simulink model "N_v6_GUI"  (R2024b)
settings: Solver=FixedStepAuto  StartTime=0.0  StopTime=solvertime  FixedStep=stepsize  RelTol=1e-3
undefined symbols (not defined in the file or in its folder): phase_delay, pulse_amp, pulse_rate
libraries: Libs_unified x1
settings Model: Creator=ball907  LastModifiedBy=ball907
settings DataIOCC: ExternalInput=params

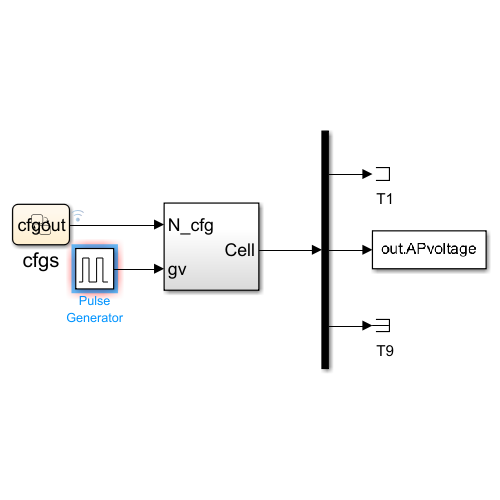
[thumbnail: Simulink's stored preview of the top-level diagram]
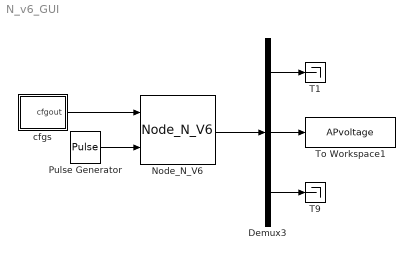
== system N_v6_GUI ==
  Demux3 : Demux  Outputs=[1, 1, 3]
  Node_N_V6 : Libs_unified/Node_N_V6  SystemSampleTime=-1  VariantActivationTime=update diagram  AllowFlexibleInterface=on  Latency=0  AutoFrameSizeCalculation=off
  Pulse Generator : DiscretePulseGenerator  PulseType=Time based  Amplitude=pulse_amp  Period=pulse_rate  PhaseDelay=phase_delay
  T1 : Terminator
  T9 : Terminator
  To Workspace1 : ToWorkspace  VariableName=APvoltage  SaveFormat=Timeseries  SampleTime=-1
  cfgs : Stateflow chart  TreatAsAtomicUnit=on
  wires:
  Demux3/2 -> To Workspace1/1
  Node_N_V6/1 -> Demux3/1
  cfgs/1(cfgout) -> Node_N_V6/1
  Pulse Generator/1 -> Node_N_V6/2
  Demux3/3 -> T9/1
  Demux3/1 -> T1/1

== stateflow chart N_v6_GUI/cfgs ==
  settings: executeAtInitialization=1
  state Ini
  (default) -> Ini : {cfgout=auto;}
  data: cfg function_output; params parameter; cfgout output
  function cfg = auto:
    | function cfg = auto
    | 
    | BCL=params(1,1);
    | SD=params(1,2);
    | f1=params(1,3);
    | f2=params(1,4);
    | sigma1sq=params(1,5);
    | sigma2sq=params(1,6);
    | 
    | d2=params(1,7); 
    | erp_out=params(1,8);
    | d0=params(1,9); 
    | MDP=params(1,10);
    | VT=params(1,11); 
    | VR=params(1,12); 
    | Vh_out=params(1,13);
    | 
    | hr_out=params(1,14); 
    | hs_out=params(1,15);
    | s_out=params(1,16);
    | j_out=params(1,17);
    | m_out=params(1,18); 
    | 
    | h_out=params(1,19);
    | f_out=params(1,20);
    | 
    | r_out=params(1,21);
    | x=params(1,22);
    | y=params(1,23);
    | 
    | cfg=[BCL, SD, f1,f2,sigma1sq, sigma2sq,d2,erp_out,d0,MDP,VT,VR,Vh_out,hr_out,hs_out,s_out,j_out,m_out,h_out,f_out,r_out,x,y];
    | end
